simulink model "Final_project"  (R2020a)
settings: Solver=ode15s  StartTime=0.0  StopTime=1.6*3600  RelTol=1e-9
values from neighbouring files (symbols this model uses):
  a = (rp + ra)/2    (= 6781)    [final_project_data.m]
  alfa_earth = alfa_earth/alfa_tot    (= 0.0757575757576)    [final_project_data.m]
  alfa_mag = alfa_mag/alfa_tot    (= 0.0151515151515)    [final_project_data.m]
  alfa_sun = alfa_sun/alfa_tot    (= 0.454545454545)    [final_project_data.m]
  e = (ra - rp)/(rp + ra)    (= 0.00147470874502)    [final_project_data.m]
  F_e = 1358    [final_project_data.m]
  G = 6.67408e-11    [final_project_data.m]
  GK = lqr(A,B,Q,R)    [final_project_data.m]
  i = 51.6    [final_project_data.m]
  I_x = I(1)    [final_project_data.m]
  I_y = I(2)    [final_project_data.m]
  I_z = I(3)    [final_project_data.m]
  m_earth = 5.972e+24    [final_project_data.m]
  mu_e = 398600    [final_project_data.m]
  n = sqrt(mu_e/a^3)    [final_project_data.m]
  omega = 0    [final_project_data.m]
  omega_e = 2*pi/T_earth    (= 7.29212351699e-05)    [final_project_data.m]
  R_e = 6371    [final_project_data.m]
  RAAN = 0    [final_project_data.m]
undefined symbols (not defined in the file or in its folder): gm, gn, gvali, hm, hn, hvali
libraries: vrlib x4, simulink_extras x3
(part 2 of 2)

== matlab function Final_project/ATTITUDE DETERMINATION/Earth Horizon Sensor/MATLAB Function ==
  data: theta input; A_epsilon output; psi input; phi input
function A_epsilon = error_matrix(theta, psi, phi)

%% Generate a random error matrix for the Sun Sensor (Lab 7)

A_epsilon = [ cos(psi)*cos(theta) cos(psi)*sin(theta)*sin(phi)+sin(psi)*cos(phi) -cos(psi)*sin(theta)*cos(phi)+sin(psi)*sin(phi)
            -sin(psi)*cos(theta)  -sin(psi)*sin(theta)*sin(phi) + cos(psi)*cos(phi) sin(psi)*sin(theta)*cos(phi) + cos(psi)*sin(phi)
            sin(theta)            -cos(theta)*sin(phi)          cos(theta)*cos(phi)];

== matlab function Final_project/ATTITUDE DETERMINATION/If Action Subsystem/MATLAB Function9 ==
  data: A input; w input; s_b input; dA output; r_n input
function dA = stateGyroObserbver(A, w, s_b,r_n)

alfa = 1*cross(s_b,A*r_n./norm(r_n));

W = [0,    -w(3),  w(2);
     w(3),   0,   -w(1);
    -w(2),  w(1),   0];

ALFA = [0,    -alfa(3),  alfa(2);
     alfa(3),   0,   -alfa(1);
    -alfa(2),  alfa(1),   0];

dA = -(ALFA+W)*A;

== matlab function Final_project/ATTITUDE DETERMINATION/Real sun sensor/MATLAB Function ==
  data: s_b input; thetas output
function thetas = SUNSENSOR(s_b)

% Direction of sun sensors
N1 = [1 0 0];
N2 = [0 1 0];
N3 = [0 0 1];

argumacos = max(min([dot(N1,s_b) dot(N2,s_b),dot(N3,s_b)],1),-1);

thetas = acos(argumacos);

== matlab function Final_project/ATTITUDE DETERMINATION/Real sun sensor/MATLAB Function1 ==
  data: thetas input; s_b output
function s_b = SUNSENSOR(thetas)

% Direction of sun sensors
N1 = [1 0 0];
N2 = [0 1 0];
N3 = [0 0 1];

cosines = cos(thetas);

N = [N1; N2; N3];

s_b = N\cosines;

== matlab function Final_project/MATLAB Function7 ==
  data: om_OBS input; domega output; omega input; I input; Md input; Mc input; alfa input
function domega = observer_gyro(om_OBS,omega,I,Md,Mc,alfa)

% Inertia moments


Ix = I(1);         %  [kg*m^2]

Iy = I(2);       %  [kg*m^2]

Iz = I(3);       %  [kg*m^2]


% Set omegas
omega_x = omega(1);
omega_y = omega(2);
omega_z = omega(3);

% Compute d_omegas 
% R -- [Km]
domega_x = (Iy - Iz)*omega_y*omega_z/Ix  + Md(1)/Ix + Mc(1)/Ix - alfa/Ix*(om_OBS(1)-omega(1));
domega_y = (Iz-Ix)*omega_x*omega_z/Iy  + Md(2)/Iy + Mc(2)/Iy - alfa /Iy * (om_OBS(2)-omega(2)); 
domega_z = (Ix - Iy)*omega_y*omega_x / Iz  + Md(3)/Iz + Mc(3)/Iz - alfa/Iz*(om_OBS(3)-omega(3));

domega = [ domega_x domega_y domega_z ];

== matlab function Final_project/MATLAB Function6 ==
  data: u input; y output
function y = DETUMBLING(u)

y = [u(1);u(2);u(3)];

== matlab function Final_project/MATLAB Function10 ==
  data: omega input; u output; J input; omegaref input; domegaref input; omegae input; Ae input; kd input; kp input
function u = NONLINCONTROL(omega,J,omegaref,domegaref,omegae,Ae,kd,kp)

skewSymm = zeros(3);
skewSymm = Ae' - Ae;
skewSymm_invhat = [-skewSymm(2,3) skewSymm(1,3) -skewSymm(1,2)]';

% u = cross(omega,J*omega) - kd*omegae - kp*J*(Ae'-Ae)
u = cross(omega,J*omega) - kd*omegae - kp*skewSymm_invhat + ...
    J*(Ae*domegaref -cross(omegae,Ae*omegaref));

== matlab function Final_project/MATLAB Function8 ==
  data: x input; dx output; omega input; omega_gyro output
function [dx, omega_gyro] = gyro(x,omega)
% Gyro param
Jz = 2e-7;
Ir = 1e-7;
omegar = 100*pi/180; %rad/s

% Tuning 
c=0.0028;
k=10;

omx = omega(1);
omy = omega(2);
omz = omega(3);

% We define the state and compute its derivatives
% angular position
th1=x(1);
th2=x(2);
th3 = x(3);
%angular rate
vax = x(4);
vay = x(5);
vaz = x(6);

dx = zeros(6,1);

dx(1)=vax;
dx(2)=vay;
dx(3)=vaz;
dx(4)= -Ir/Jz*omegar*omx - c/Jz*vax - k/Jz*th1;
dx(5)= -Ir/Jz*omegar*omy - c/Jz*vay - k/Jz*th2;
dx(6)= -Ir/Jz*omegar*omz - c/Jz*vaz - k/Jz*th3;

omega_gyro = -k*[th1 th2 th3]./(Ir*omegar);

== matlab function Final_project/MATLAB Function11 ==
  data: A input size=[3 3]; A_orthonormal output size=[3 3]
function A_orthonormal = orthonormilizer(A)

% Iterative formulas for orthonormalization
% first order approximation: single step iteration
A_orthonormal = A*3/2 - A*(A')*A/2;

end

== matlab function Final_project/MATLAB Function ==
  data: omega input; I input; domega output; Md input; Mc input
function domega = euler_equations(omega,I,Md,Mc)

% Inertia moments


Ix = I(1);         %  [kg*m^2]

Iy = I(2);       %  [kg*m^2]

Iz = I(3);       %  [kg*m^2]


% Set omegas
omega_x = omega(1);
omega_y = omega(2);
omega_z = omega(3);

% Compute d_omegas with gravity gradient torque
% R -- [Km]
domega_x = (Iy - Iz)*omega_y*omega_z/Ix  + Md(1)/Ix + Mc(1)/Ix;
domega_y = (Iz-Ix)*omega_x*omega_z/Iy  + Md(2)/Iy + Mc(2)/Iy;
domega_z = (Ix - Iy)*omega_y*omega_x / Iz  + Md(3)/Iz + Mc(3)/Iz;

domega = [ domega_x domega_y domega_z ];
end

== matlab function Final_project/ATTITUDE DETERMINATION/QUEST Attitude Determination/MATLAB Function1 ==
  data: B input size=[3 3]; Abn output size=[3 3]
function Abn= SVD(B)


[U,S,V] = svd(B);

M = diag([1 1 det(U)*det(V)]);
Abn = U*M*V';

== matlab function Final_project/FULL STATE FEEDBACK CONTROLLER ==
  data: A_e input; u_id output size=3; omega_e input; GK input
function u_id = LQR(A_e,omega_e,GK)

alfaz = A_e(1,2);
alfay = A_e(3,1);
alfax = A_e(2,3);

dalfax = omega_e(1);
dalfay = omega_e(2);
dalfaz = omega_e(3);

statevec = [alfax alfay alfaz dalfax dalfay dalfaz]';

u_id = -GK*statevec;

== matlab function Final_project/MATLAB Function1 ==
  data: omega input; qdot output; q input
function qdot = kyn_quat(omega,q)

% Kinematics using quaternions

W = [0 omega(3) -omega(2) omega(1)
    -omega(3) 0 omega(1) omega(2)
    omega(2) -omega(1) 0 omega(3)
    - omega(1) -omega(2) -omega(3) 0];

qdot = 1/2 * W *q;
end

== matlab function Final_project/CMG actuator/MATLAB Function ==
  data: delta input; B output; beta input; omega_r input; Ir input; h_CMG output; nullCOMMAND output size=4 [..1]
function [B,h_CMG,nullCOMMAND]  = CMG(delta,beta,omega_r,Ir)
% Function that computes the B matrix of a 4 CMG system with a pyramid
% shape, with sides inclined of an angle beta 
% delta: gimbal angle vector of the Control Moment Gyros [rad]
% beta: gimbal mounting angle                            [rad]
% omega_r: spin rate of the CMGs                         [rad/s]
% Ir: inertia moment of each wheel

hr = omega_r*Ir;
B = hr.*[-cos(beta)*cos(delta(1))   sin(delta(2))   cos(beta)*cos(delta(3)) -sin(delta(4));
    -sin(delta(1))  -cos(beta)*cos(delta(2))    sin(delta(3))   cos(beta)*cos(delta(4));
    sin(beta)*cos(delta(1)) sin(beta)*cos(delta(2)) sin(beta)*cos(delta(3)) sin(beta)*cos(delta(4));];

% attitude matrix of the CMGs
A = [-cos(beta)*sin(delta(1))   -cos(delta(2))  cos(beta)*sin(delta(3)) cos(delta(4));
    cos(delta(1))   -cos(beta)*sin(delta(2))    -cos(delta(3))  cos(beta)*sin(delta(4));
    sin(beta)*sin(delta(1))   sin(beta)*sin(delta(2)) sin(beta)*sin(delta(3))   sin(beta)*sin(delta(4));];

%  Total angular momentum vector of CMG
h_CMG = hr.*A*[1;1;1;1;];

% Compute the null space of matrix B, for the null motion command
nullCOMMAND = zeros(4,1);
nullCOMMAND = nullCOMMAND + null(B);

== matlab function Final_project/Matrix A_B//L/MATLAB Function3 ==
  data: theta input; A_LN output; i input; w input; RAAN input
function A_LN = matrixA_LN(theta,i,w,RAAN)

% i - orbital inclination [rad]
% theta - true anomaly    [rad]

A_LN_3 = [cos(theta+w)    sin(theta+w)    0
        -sin(theta+w)   cos(theta+w)    0
        0           0           1];
    
A_LN_2 = [1     0       0
        0   cos(i)  sin(i)
        0   -sin(i) cos(i)];
    
A_LN_1 = [cos(RAAN)    sin(RAAN)    0
        -sin(RAAN)   cos(RAAN)    0
        0           0           1];
% Rotation matrix to reach the orbital frame
    
A_LN = A_LN_3 * A_LN_2 *A_LN_1;

== matlab function Final_project/Approximate orbit model/orbit model - S//C orbit wrt Earth/MATLAB Function4 ==
  data: n input; theta_dot output; e input; theta input
function theta_dot = propagator(n,e,theta)

% n - n_Earth

theta_dot = n*(1+e*cos(theta))^2/(1-e^2)^(3/2) ;

== matlab function Final_project/MATLAB Function3 ==
  data: q input; Abn output
function Abn = fcn(q)

Abn = [q(1)^2-q(2)^2-q(3)^2+q(4)^2  2*(q(1)*q(2)+q(3)*q(4))         2*(q(1)*q(3)-q(2)*q(4))
        2*(q(1)*q(2)-q(3)*q(4))     -q(1)^2+q(2)^2-q(3)^2+q(4)^2    2*(q(2)*q(3)+q(1)*q(4))
        2*(q(1)*q(3)+q(2)*q(4))     2*(q(2)*q(3)-q(1)*q(4))         -q(1)^2-q(2)^2+q(3)^2+q(4)^2];
    
end

== matlab function Final_project/Approximate orbit model/MATLAB Function3 ==
  data: vector input; versor output
function versor = nromalize(vector)

versor = vector./norm(vector);

== matlab function Final_project/MATLAB Function13 ==
  data: A_est input; A_raw input; w input; y output; alpha1 input
function y = stateObserbver(A_est, A_raw, w, alpha1)


W = [0,    -w(3),  w(2);
     w(3),   0,   -w(1);
    -w(2),  w(1),   0];


A_est_dot = -W * A_est + alpha1*(A_est-A_raw);


y = A_est_dot;
